simulink model "sampleModel1512_2_sub_sub_sub"  (R2023a)
settings: Solver=VariableStepAuto  StartTime=0.0  StopTime=10.0  RelTol=1e-3
libraries: hdlsllib x7, simulink x2
settings Model: Creator=user1  LastModifiedBy=user1
settings OptimizationCC: BlockReduction=off  ConditionallyExecuteInputs=off

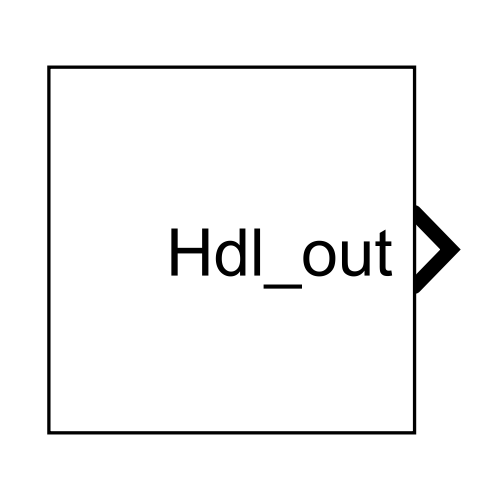
[thumbnail: Simulink's stored preview of the top-level diagram]
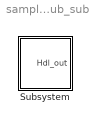
== system sampleModel1512_2_sub_sub_sub ==
  Subsystem : Subsystem

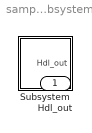
== system sampleModel1512_2_sub_sub_sub/Subsystem ==
  Subsystem : Subsystem
  Hdl_out : Outport  OutDataTypeStr=uint8

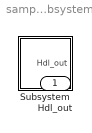
== system sampleModel1512_2_sub_sub_sub/Subsystem/Subsystem ==
  Subsystem : Subsystem
  Hdl_out : Outport  OutDataTypeStr=uint8

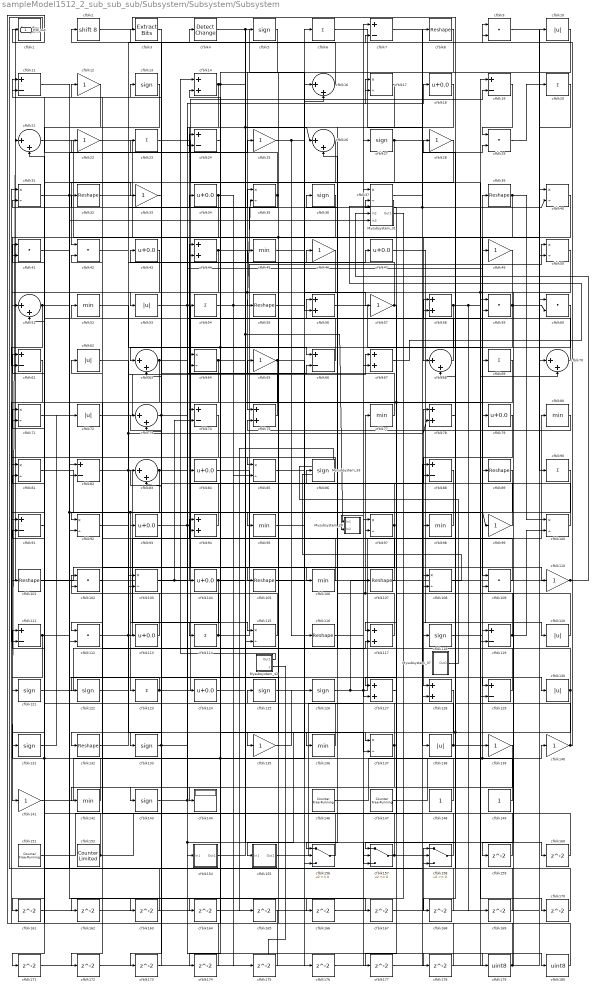
== system sampleModel1512_2_sub_sub_sub/Subsystem/Subsystem/Subsystem ==
  Mysubsystem_28 : Subsystem  TreatAsAtomicUnit=on  RTWFcnName=Mysubsystem_28
      settings: RTWFcnNameOpts=User specified  RTWFileNameOpts=Use function name
  Mysubsystem_31 : Subsystem  TreatAsAtomicUnit=on  RTWFcnName=Mysubsystem_31
      settings: RTWFcnNameOpts=User specified  RTWFileNameOpts=Use function name
  Mysubsystem_33 : Subsystem  TreatAsAtomicUnit=on  RTWFcnName=Mysubsystem_33
      settings: RTWFcnNameOpts=User specified  RTWFileNameOpts=Use function name
  Mysubsystem_37 : Subsystem  TreatAsAtomicUnit=on  RTWFcnName=Mysubsystem_37
      settings: RTWFcnNameOpts=User specified  RTWFileNameOpts=Use function name
  Mysubsystem_42 : Subsystem  TreatAsAtomicUnit=on  RTWFcnName=Mysubsystem_42
      settings: RTWFcnNameOpts=User specified  RTWFileNameOpts=Use function name
  cfblk1 : hdlsllib/Logic and Bit Operations/Detect Rise Nonnegative  vinit=0  OutDataTypeStr=uint8
  cfblk{10,53,62,72,120,130,138} (7 alike) : Abs  OutDataTypeStr=uint8  SaturateOnIntegerOverflow=off
  cfblk{17,31,35,37,40,50,64,71,81,85,92,97,100,103,108,115,137} (17 alike) : Product  Inputs=*/  OutDataTypeStr=uint8  RndMeth=Zero  SaturateOnIntegerOverflow=on
  cfblk{8,32,39,55,89,101,105,107,116,132} (10 alike) : Reshape
  cfblk{9,29,41..42,59..60,102,109,112} (9 alike) : DotProduct  OutDataTypeStr=uint8
  cfblk{18,34,43,47,79,84,93,104,113,124} (10 alike) : Bias  Bias=0.0  SaturateOnIntegerOverflow=off
  cfblk{45,52,77,80,95,98,106,136,142} (9 alike) : MinMax  OutDataTypeStr=uint8
  cfblk{7,11,19,24,61,66,74,82,88,91,111,119,129} (13 alike) : Sum  Inputs=+-  OutDataTypeStr=uint8
  cfblk{12,22,25,28,33,46,49,57,65,99,110,135,139..141} (15 alike) : Gain  OutDataTypeStr=uint8
  cfblk{6,20,23,54,69,90,114,123} (8 alike) : Sum  Inputs=+  OutDataTypeStr=uint8
  cfblk{14,44,56,58,67,75,78,94,117,127..128} (11 alike) : Sum  OutDataTypeStr=uint8
  cfblk{5,13,27,36,86,118,121..122,125..126,131,133,143} (13 alike) : Signum
  cfblk144 : Display
  cfblk146 : hdlsllib/Sources/Counter Free-Running  NumBits=16  tsamp=-1
  cfblk147 : hdlsllib/Sources/Counter Free-Running  NumBits=16  tsamp=-1
  cfblk148 : Constant  OutDataTypeStr=uint8  SampleTime=-1
  cfblk149 : Constant  OutDataTypeStr=uint8  SampleTime=-1
  cfblk151 : hdlsllib/Sources/Counter Free-Running  NumBits=16  tsamp=-1
  cfblk152 : hdlsllib/Sources/Counter Limited  uplimit=7  tsamp=-1
  cfblk154 : Subsystem
      settings: LibrarySourceBlock=|
      | hdlsllib/Ports &
      | Subsystems/Subsystem
  cfblk155 : Subsystem
      settings: LibrarySourceBlock=|
      | hdlsllib/Ports &
      | Subsystems/Subsystem
  cfblk156 : Switch  OutDataTypeStr=uint8  SaturateOnIntegerOverflow=off  InputSameDT=off
  cfblk157 : Switch  OutDataTypeStr=uint8  SaturateOnIntegerOverflow=off  InputSameDT=off
  cfblk158 : Switch  OutDataTypeStr=uint8  SaturateOnIntegerOverflow=off  InputSameDT=off
  cfblk{159..178} (20 alike) : Delay  SampleTime=1
  cfblk{16,21,26,51,63,68,70,73,83} (9 alike) : Sum  Inputs=|++  OutDataTypeStr=uint8
  cfblk179 : DataTypeConversion  OutDataTypeStr=uint8  SaturateOnIntegerOverflow=off  RndMeth=Floor
  cfblk180 : DataTypeConversion  OutDataTypeStr=uint8  SaturateOnIntegerOverflow=off  RndMeth=Floor
  cfblk2 : ArithShift  BitShiftNumber=8
  cfblk3 : simulink/Logic and Bit Operations/Extract Bits  bitsToExtract=Upper half  numBits=8  bitIdxRange=[0 7]  outScalingMode=Preserve fixed-point scaling
      settings: LibrarySourceBlock=|
      | hdlsllib/Logic and Bit
      | Operations/Extract Bits
  cfblk4 : simulink/Logic and Bit Operations/Detect Change  vinit=0  OutDataTypeStr=uint8
      settings: LibrarySourceBlock=|
      | hdlsllib/Logic and Bit
      | Operations/Detect
      | Change
  Hdl_out : Outport  OutDataTypeStr=uint8
  wires:
  cfblk29/1 -> cfblk20/1
  cfblk83/1 -> cfblk59/2, cfblk103/2, cfblk123/1
  cfblk142/1 -> cfblk81/2, cfblk21/1
  cfblk35/1 -> cfblk31/2, cfblk11/1
  cfblk8/1 -> cfblk132/1
  cfblk2/1 -> cfblk157/1
  cfblk135/1 -> cfblk126/1
  cfblk117/1 -> cfblk26/2, cfblk77/1
  cfblk140/1 -> cfblk88/2, cfblk9/1
  cfblk72/1 -> cfblk67/1
  cfblk114/1 -> cfblk102/1, cfblk50/1
  cfblk77/1 -> cfblk11/2
  cfblk43/1 -> cfblk53/1
  cfblk82/1 -> cfblk137/2, cfblk115/1
  cfblk98/1 -> cfblk92/1
  cfblk39/1 -> cfblk100/1, cfblk141/1
  cfblk147/1 -> cfblk10/1, cfblk39/1
  cfblk79/1 -> cfblk128/1
  cfblk34/1 -> cfblk85/2, cfblk143/1
  cfblk118/1 -> cfblk119/1
  cfblk56/1 -> cfblk109/1
  cfblk70/1 -> cfblk21/2
  cfblk128/1 -> cfblk155/1(In1)
  cfblk36/1 -> cfblk85/1, cfblk93/1
  cfblk84/1 -> cfblk106/1
  cfblk24/1 -> cfblk144/1
  cfblk47/1 -> cfblk119/2
  cfblk123/1 -> cfblk122/1, cfblk19/2
  cfblk5/1 -> cfblk75/1
  cfblk126/1 -> cfblk107/1, cfblk80/1, Mysubsystem_28/2(In2)
  cfblk125/1 -> cfblk179/1
  cfblk97/1 -> cfblk142/1, cfblk73/1
  cfblk131/1 -> cfblk72/1
  cfblk27/1 -> cfblk29/2, cfblk42/1
  cfblk94/1 -> cfblk43/1
  cfblk17/1 -> cfblk104/1
  cfblk21/1 -> cfblk69/1
  cfblk69/1 -> cfblk71/2, cfblk117/1
  cfblk154/1(Out1) -> Mysubsystem_28/1(In1), cfblk56/1
  cfblk112/1 -> cfblk89/1, cfblk9/2, cfblk78/2
  cfblk103/1 -> cfblk74/2, cfblk130/1
  cfblk89/1 -> cfblk127/1
  cfblk104/1 -> cfblk173/1, cfblk18/1
  cfblk11/1 -> cfblk92/2
  cfblk53/1 -> cfblk49/1, cfblk110/1
  cfblk111/1 -> cfblk121/1, Mysubsystem_31/3(In3)
  cfblk143/1 -> cfblk65/1, cfblk178/1, cfblk156/3
  cfblk116/1 -> cfblk27/1
  cfblk62/1 -> cfblk103/1
  cfblk156/1 -> cfblk52/1
  cfblk22/1 -> cfblk90/1
  cfblk40/1 -> cfblk68/1
  cfblk88/1 -> cfblk135/1
  cfblk31/1 -> cfblk167/1, cfblk33/1
  cfblk42/1 -> cfblk35/1
  cfblk68/1 -> cfblk44/1
  cfblk14/1 -> cfblk24/2, cfblk74/1, cfblk79/1
  cfblk74/1 -> cfblk101/1
  cfblk26/1 -> cfblk115/2
  cfblk20/1 -> cfblk50/2
  cfblk130/1 -> cfblk36/1, cfblk174/1, cfblk168/1
  cfblk80/1 -> cfblk75/2
  cfblk122/1 -> cfblk47/1
  cfblk33/1 -> cfblk113/1
  cfblk66/1 -> cfblk23/1
  cfblk16/1 -> cfblk2/1
  cfblk41/1 -> cfblk25/1
  cfblk115/1 -> cfblk12/1
  cfblk151/1 -> cfblk98/1
  cfblk155/1(Out1) -> cfblk67/2
  cfblk146/1 -> cfblk118/1
  cfblk101/1 -> cfblk108/1
  cfblk92/1 -> cfblk4/1
  cfblk37/1 -> cfblk129/1, cfblk40/2
  cfblk119/1 -> cfblk100/2, cfblk28/1
  cfblk149/1 -> cfblk94/2, cfblk61/1
  cfblk148/1 -> cfblk94/1, cfblk83/1
  cfblk106/1 -> cfblk42/2
  cfblk129/1 -> cfblk32/1
  cfblk75/1 -> cfblk54/1
  cfblk100/1 -> cfblk86/1
  cfblk44/1 -> cfblk82/2, cfblk8/1
  cfblk32/1 -> cfblk154/1(In1)
  cfblk90/1 -> cfblk136/1
  cfblk86/1 -> cfblk84/1
  cfblk58/1 -> cfblk170/1, cfblk169/1, cfblk114/1, cfblk63/2
  cfblk6/1 -> cfblk138/1
  cfblk18/1 -> cfblk156/1
  cfblk81/1 -> cfblk124/1
  cfblk4/1 -> cfblk56/2, cfblk108/2, cfblk26/1
  cfblk152/1 -> cfblk5/1, cfblk111/1
  cfblk1/1 -> cfblk158/1
  cfblk93/1 -> cfblk17/2, cfblk78/1
  cfblk51/1 -> cfblk128/2, cfblk61/2
  cfblk52/1 -> cfblk66/1
  cfblk71/1 -> cfblk166/1, cfblk99/1
  cfblk85/1 -> cfblk17/1
  cfblk141/1 -> cfblk16/1
  cfblk109/1 -> cfblk46/1
  cfblk78/1 -> cfblk58/1
  cfblk57/1 -> cfblk13/1, cfblk137/1
  cfblk3/1 -> cfblk63/1
  cfblk64/1 -> cfblk161/1, cfblk160/1
  cfblk73/1 -> cfblk58/2, cfblk133/1
  cfblk65/1 -> cfblk157/3, cfblk112/1
  cfblk7/1 -> cfblk120/1
  cfblk63/1 -> cfblk171/1, cfblk66/2
  cfblk12/1 -> cfblk131/1
  cfblk13/1 -> cfblk112/2
  cfblk45/1 -> cfblk7/2
  cfblk158/1 -> cfblk97/2
  cfblk28/1 -> cfblk91/1
  cfblk113/1 -> cfblk62/1
  cfblk124/1 -> cfblk117/2
  cfblk107/1 -> cfblk24/1
  cfblk120/1 -> cfblk37/2
  cfblk102/1 -> cfblk22/1
  cfblk9/1 -> cfblk70/1
  cfblk55/1 -> cfblk57/1
  cfblk91/1 -> cfblk41/1
  cfblk60/1 -> cfblk95/1
  cfblk157/1 -> cfblk102/2, cfblk140/1
  cfblk54/1 -> cfblk175/1, cfblk35/2
  cfblk59/1 -> cfblk105/1, cfblk51/1, cfblk60/2
  cfblk10/1 -> cfblk64/1
  cfblk121/1 -> cfblk16/2
  cfblk105/1 -> cfblk127/2
  cfblk138/1 -> cfblk70/2, cfblk45/1
  cfblk99/1 -> cfblk14/2
  cfblk137/1 -> cfblk163/1, cfblk51/2
  cfblk133/1 -> cfblk156/2, cfblk83/2
  cfblk136/1 -> cfblk71/1
  cfblk49/1 -> cfblk129/2, cfblk55/1, cfblk81/1
  cfblk25/1 -> cfblk116/1, cfblk6/1
  cfblk61/1 -> cfblk111/2
  cfblk23/1 -> cfblk139/1
  cfblk132/1 -> cfblk64/2
  cfblk19/1 -> cfblk29/1
  cfblk50/1 -> cfblk159/1
  cfblk159/1 -> cfblk19/1
  cfblk160/1 -> cfblk44/2
  cfblk161/1 -> cfblk158/3
  cfblk162/1 -> cfblk97/1
  cfblk163/1 -> cfblk82/1
  cfblk46/1 -> cfblk164/1
  cfblk164/1 -> cfblk158/2
  cfblk165/1 -> cfblk1/1
  cfblk166/1 -> cfblk157/2
  cfblk167/1 -> cfblk40/1
  cfblk168/1 -> cfblk7/1
  cfblk169/1 -> cfblk68/2
  cfblk170/1 -> cfblk41/2
  cfblk171/1 -> cfblk88/1
  cfblk139/1 -> cfblk172/1
  cfblk172/1 -> cfblk37/1
  cfblk173/1 -> cfblk73/2
  cfblk174/1 -> cfblk31/1
  cfblk175/1 -> cfblk91/2
  cfblk95/1 -> cfblk176/1
  cfblk176/1 -> cfblk60/1
  cfblk127/1 -> cfblk177/1
  cfblk177/1 -> cfblk59/1
  cfblk178/1 -> cfblk34/1
  cfblk179/1 -> cfblk3/1, cfblk109/2
  cfblk180/1 -> cfblk125/1
  cfblk67/1 -> Mysubsystem_31/1(In1)
  cfblk110/1 -> Hdl_out/1, Mysubsystem_31/2(In2)
  Mysubsystem_31/1(Out1) -> cfblk162/1
  cfblk108/1 -> Mysubsystem_33/2(In2)
  Mysubsystem_33/1(Out1) -> cfblk165/1
  Mysubsystem_37/1(Out1) -> Mysubsystem_33/1(In1)
  Mysubsystem_42/1(Out1) -> cfblk14/1
  Mysubsystem_42/2(y) -> cfblk180/1

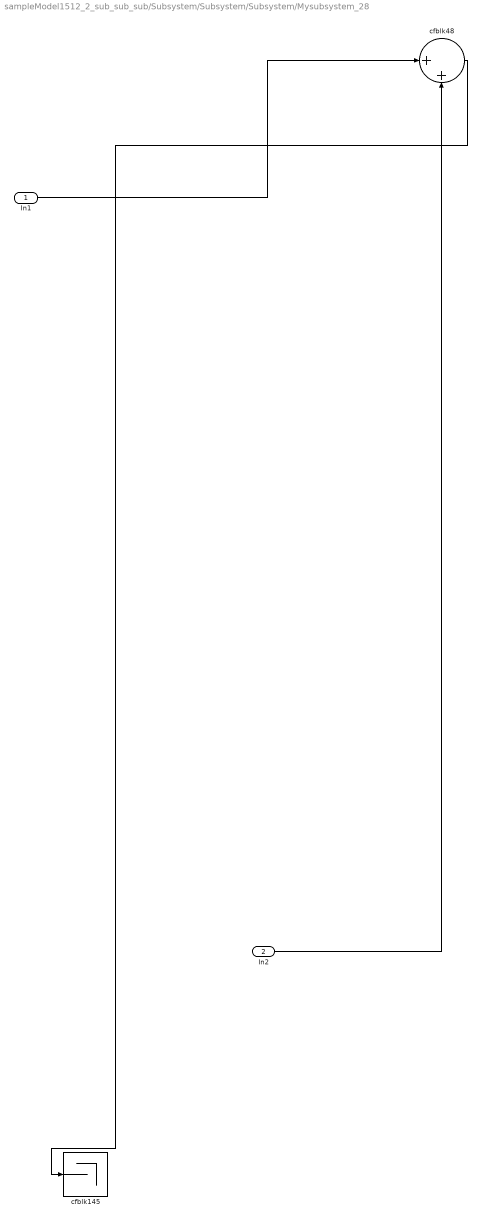
== system sampleModel1512_2_sub_sub_sub/Subsystem/Subsystem/Subsystem/Mysubsystem_28 ==
  In1 : Inport
  In2 : Inport  Port=2
  cfblk145 : Terminator
  cfblk48 : Sum  Inputs=|++
  wires:
  In1/1 -> cfblk48/1
  In2/1 -> cfblk48/2
  cfblk48/1 -> cfblk145/1

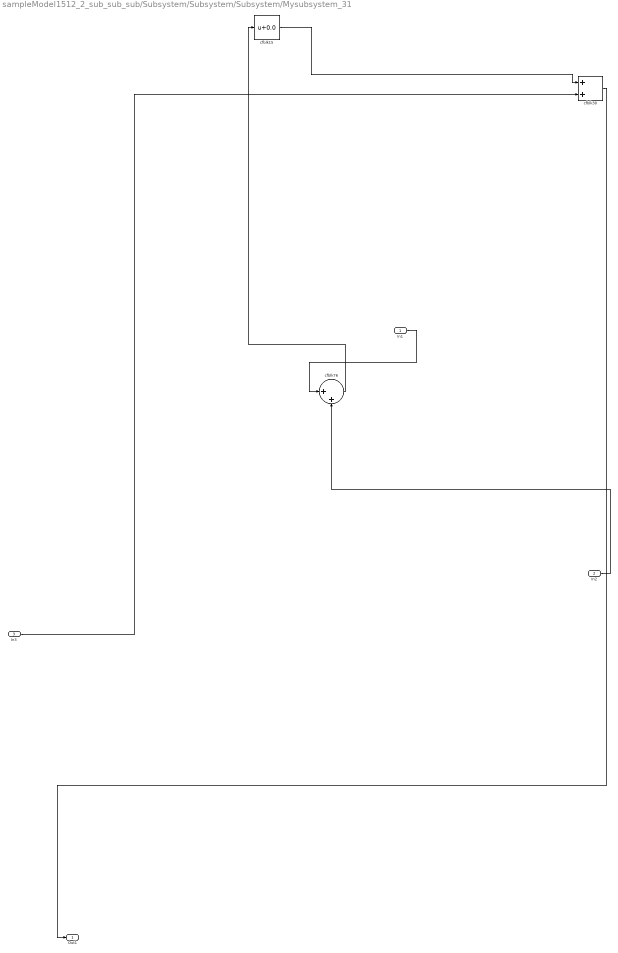
== system sampleModel1512_2_sub_sub_sub/Subsystem/Subsystem/Subsystem/Mysubsystem_31 ==
  In1 : Inport
  In2 : Inport  Port=2
  In3 : Inport  Port=3
  cfblk15 : Bias  Bias=0.0  SaturateOnIntegerOverflow=off
  cfblk30 : Sum
  cfblk76 : Sum  Inputs=|++
  Out1 : Outport
  wires:
  cfblk30/1 -> Out1/1
  In1/1 -> cfblk76/1
  In2/1 -> cfblk76/2
  In3/1 -> cfblk30/2
  cfblk15/1 -> cfblk30/1
  cfblk76/1 -> cfblk15/1

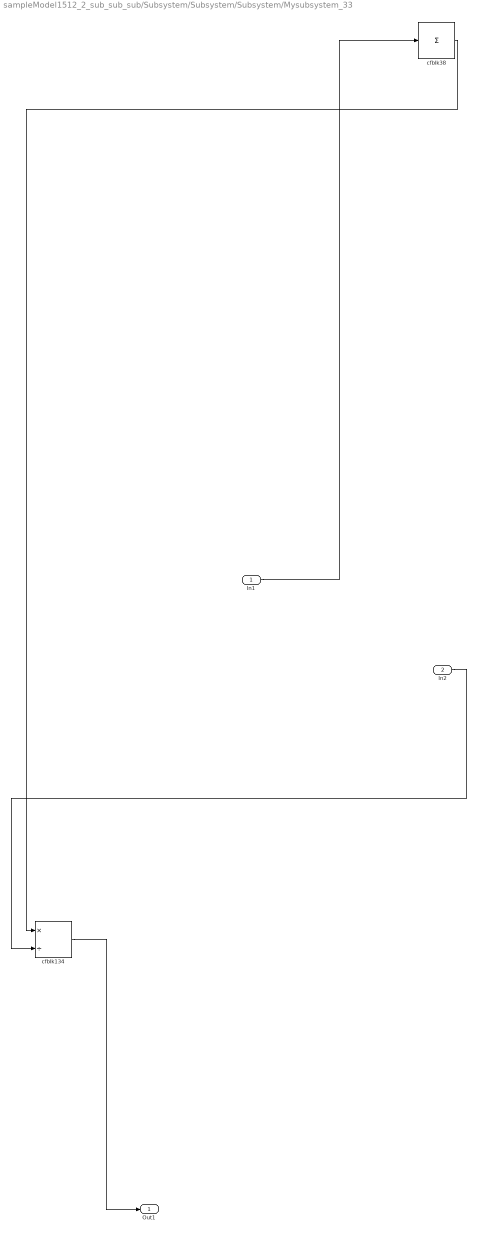
== system sampleModel1512_2_sub_sub_sub/Subsystem/Subsystem/Subsystem/Mysubsystem_33 ==
  In1 : Inport
  In2 : Inport  Port=2
  cfblk134 : Product  Inputs=*/  RndMeth=Zero  SaturateOnIntegerOverflow=on
  cfblk38 : Sum  Inputs=+
  Out1 : Outport
  wires:
  In1/1 -> cfblk38/1
  cfblk134/1 -> Out1/1
  In2/1 -> cfblk134/2
  cfblk38/1 -> cfblk134/1

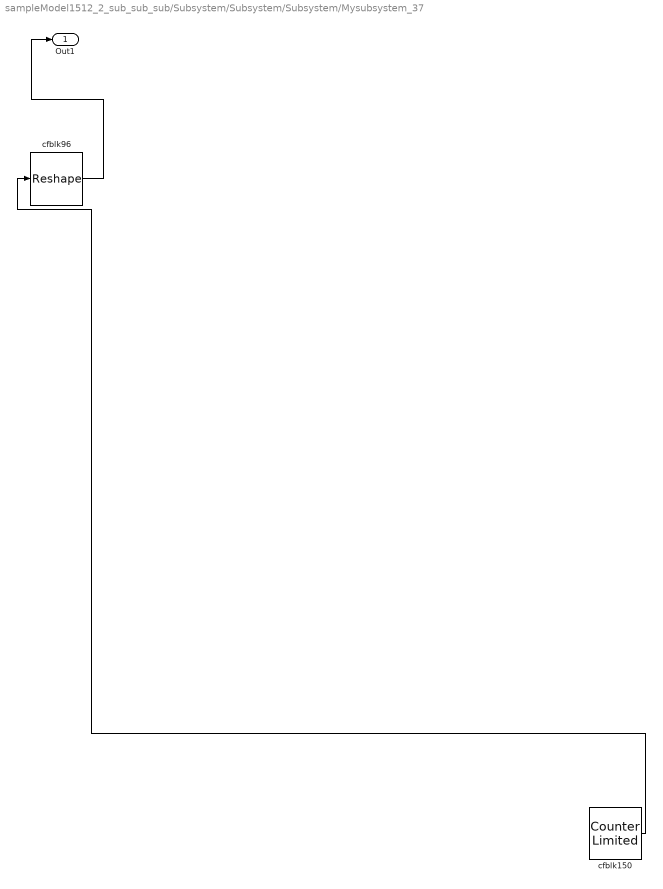
== system sampleModel1512_2_sub_sub_sub/Subsystem/Subsystem/Subsystem/Mysubsystem_37 ==
  cfblk150 : hdlsllib/Sources/Counter Limited  uplimit=7  tsamp=-1
  cfblk96 : Reshape
  Out1 : Outport
  wires:
  cfblk96/1 -> Out1/1
  cfblk150/1 -> cfblk96/1

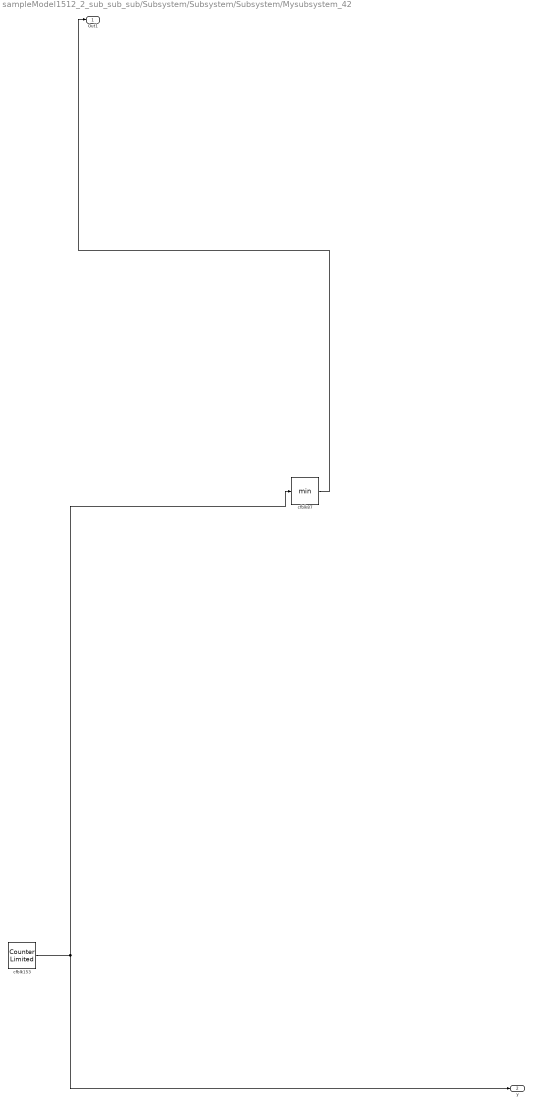
== system sampleModel1512_2_sub_sub_sub/Subsystem/Subsystem/Subsystem/Mysubsystem_42 ==
  cfblk153 : hdlsllib/Sources/Counter Limited  uplimit=7  tsamp=-1
  cfblk87 : MinMax
  Out1 : Outport
  y : Outport  Port=2
  wires:
  cfblk87/1 -> Out1/1
  cfblk153/1 -> cfblk87/1, y/1

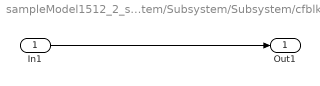
== system sampleModel1512_2_sub_sub_sub/Subsystem/Subsystem/Subsystem/cfblk154 ==
  In1 : Inport
  Out1 : Outport
  wires:
  In1/1 -> Out1/1

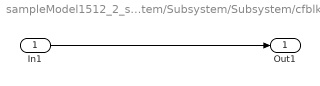
== system sampleModel1512_2_sub_sub_sub/Subsystem/Subsystem/Subsystem/cfblk155 ==
  In1 : Inport
  Out1 : Outport
  wires:
  In1/1 -> Out1/1
